simulink library "ESSLibrary"  (R2020a)
settings: Solver=VariableStepAuto  StartTime=0.0  StopTime=10.0  RelTol=1e-3
libraries: $bdroot x82, powerlib_meascontrol x10, simulink x7
(part 6 of 7)

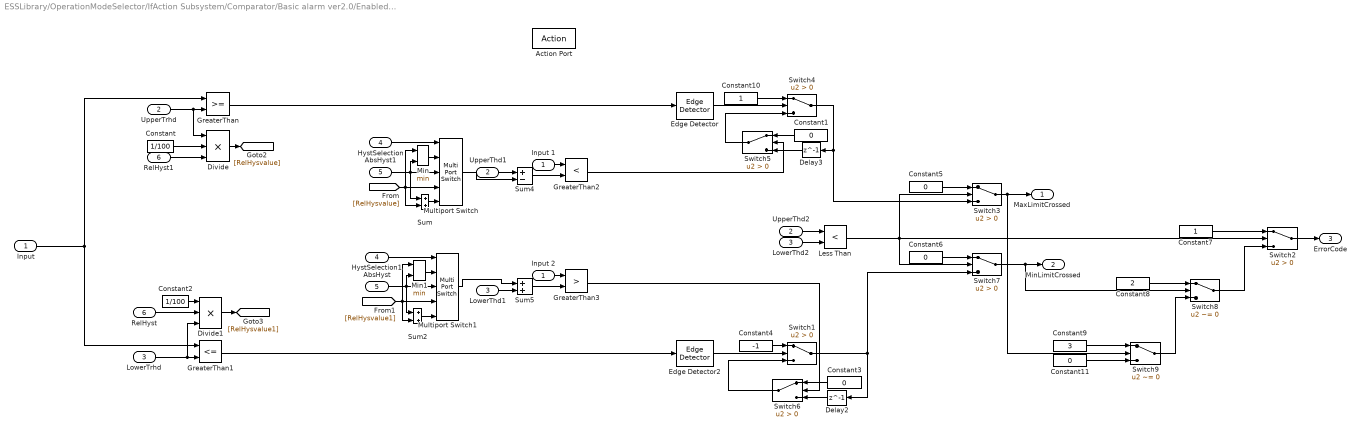
== system ESSLibrary/OperationModeSelector/IfAction Subsystem/Comparator/Basic alarm ver2.0/Enabled Subsystem1 ==
  "Input " : Inport
  UpperTrhd : Inport  Port=2
  LowerTrhd : Inport  Port=3
  HystSelection : Inport  Port=4
  AbsHyst : Inport  Port=5
  RelHyst : Inport  Port=6
  Action Port : ActionPort
  AbsHyst1 : InportShadow  Port=5
  Constant : Constant  Value=1/100  SampleTime=-1
  Constant1 : Constant  Value=0  OutDataTypeStr=int8  SampleTime=-1
  Constant10 : Constant  OutDataTypeStr=int8  SampleTime=-1
  Constant11 : Constant  Value=0  OutDataTypeStr=int64  SampleTime=-1
  Constant2 : Constant  Value=1/100  SampleTime=-1
  Constant3 : Constant  Value=0  OutDataTypeStr=int8  SampleTime=-1
  Constant4 : Constant  Value=-1  OutDataTypeStr=int8  SampleTime=-1
  Constant5 : Constant  Value=0  OutDataTypeStr=boolean  SampleTime=-1
  Constant6 : Constant  Value=0  OutDataTypeStr=boolean  SampleTime=-1
  Constant7 : Constant  OutDataTypeStr=int64  SampleTime=-1
  Constant8 : Constant  Value=2  OutDataTypeStr=int64  SampleTime=-1
  Constant9 : Constant  Value=3  OutDataTypeStr=int64  SampleTime=-1
  Delay2 : Delay  DelayLength=1  InitialCondition=0
  Delay3 : Delay  DelayLength=1  InitialCondition=0
  Divide : Product  Inputs=***
  Divide1 : Product  Inputs=***
  Edge Detector : powerlib_meascontrol/Logic/Edge Detector  model=Rising  ic=0  Ts=-1
      settings: SourceProductBaseCode=PS
  Edge Detector2 : powerlib_meascontrol/Logic/Edge Detector  model=Rising  ic=0  Ts=-1
      settings: SourceProductBaseCode=PS
  GreaterThan : RelationalOperator  OutDataTypeStr=boolean  RndMeth=Simplest
  GreaterThan1 : RelationalOperator  Operator=<=  OutDataTypeStr=boolean  RndMeth=Simplest
  GreaterThan2 : RelationalOperator  Operator=<  OutDataTypeStr=boolean  RndMeth=Simplest
  GreaterThan3 : RelationalOperator  Operator=>  OutDataTypeStr=boolean  RndMeth=Simplest
  HystSelection1 : InportShadow  Port=4
  Input 1 : InportShadow
  Input 2 : InportShadow
  Less Than : RelationalOperator  Operator=<  OutDataTypeStr=boolean  RndMeth=Simplest
  LowerThd1 : InportShadow  Port=3
  LowerThd2 : InportShadow  Port=3
  Min : MinMax  Inputs=2
  Min1 : MinMax  Inputs=2
  Multiport Switch : MultiPortSwitch  Inputs=4
  Multiport Switch1 : MultiPortSwitch  Inputs=4
  RelHyst1 : InportShadow  Port=6
  Sum : Sum
  Sum2 : Sum
  Sum4 : Sum  Inputs=+-
  Sum5 : Sum
  Switch{1..7} (7 alike) : Switch  Criteria=u2 > Threshold
  Switch8 : Switch  Criteria=u2 ~= 0
  Switch9 : Switch  Criteria=u2 ~= 0
  UpperThd1 : InportShadow  Port=2
  UpperThd2 : InportShadow  Port=2
  MaxLimitCrossed : Outport
  MinLimitCrossed : Outport  Port=2
  ErrorCode : Outport  Port=3  OutDataTypeStr=int64
  wires:
  Constant4/1 -> Switch1/1
  GreaterThan/1 -> Edge Detector/1
  "Input "/1 -> GreaterThan/1, GreaterThan1/1
  UpperTrhd/1 -> Divide/1, GreaterThan/2
  LowerTrhd/1 -> Divide1/3, GreaterThan1/2
  HystSelection/1 -> Multiport Switch/1
  AbsHyst1/1 -> Min/2, Sum/1, Multiport Switch/3
  [RelHysvalue] -> Min/1, Sum/2, Multiport Switch/4
  Sum/1 -> Multiport Switch/5
  Divide/1 -> [RelHysvalue]
  Min/1 -> Multiport Switch/2
  Input 1/1 -> GreaterThan2/1
  Constant10/1 -> Switch4/1
  Edge Detector/1 -> Switch4/2
  Switch5/1 -> Switch4/3
  Switch4/1 -> Switch3/3, Delay3/1
  Constant/1 -> Divide/2
  RelHyst1/1 -> Divide/3
  RelHyst/1 -> Divide1/2
  Constant2/1 -> Divide1/1
  Divide1/1 -> [RelHysvalue1]
  HystSelection1/1 -> Multiport Switch1/1
  Min1/1 -> Multiport Switch1/2
  AbsHyst/1 -> Sum2/1, Min1/2, Multiport Switch1/3
  [RelHysvalue1] -> Sum2/2, Multiport Switch1/4, Min1/1
  Sum2/1 -> Multiport Switch1/5
  Input 2/1 -> GreaterThan3/1
  GreaterThan1/1 -> Edge Detector2/1
  Edge Detector2/1 -> Switch1/2
  Switch6/1 -> Switch1/3
  GreaterThan3/1 -> Switch6/2
  Sum4/1 -> GreaterThan2/2
  Multiport Switch/1 -> Sum4/2
  UpperThd1/1 -> Sum4/1
  Sum5/1 -> GreaterThan3/2
  Multiport Switch1/1 -> Sum5/1
  LowerThd1/1 -> Sum5/2
  GreaterThan2/1 -> Switch5/2
  Constant1/1 -> Switch5/1
  Constant3/1 -> Switch6/1
  Delay3/1 -> Switch5/3
  Delay2/1 -> Switch6/3
  Switch3/1 -> Switch9/2, MaxLimitCrossed/1
  Less Than/1 -> Switch2/2, Switch3/2, Switch7/2
  Constant5/1 -> Switch3/1
  Switch1/1 -> Switch7/3, Delay2/1
  Constant6/1 -> Switch7/1
  Switch7/1 -> Switch8/2, MinLimitCrossed/1
  Switch8/1 -> Switch2/3
  Constant7/1 -> Switch2/1
  Switch2/1 -> ErrorCode/1
  LowerThd2/1 -> Less Than/2
  UpperThd2/1 -> Less Than/1
  Constant8/1 -> Switch8/1
  Constant9/1 -> Switch9/1
  Constant11/1 -> Switch9/3
  Switch9/1 -> Switch8/3

== system ESSLibrary/PFReference_P/If Action Subsystem/Safe Divider/Subsystem/Subsystem21 ==
  Denominator : Inport  OutDataTypeStr=double
  Compare To Zero : simulink/Logic and Bit Operations/Compare To Zero  relop===  OutDataTypeStr=boolean
  Constant : Constant  Value=0  SampleTime=-1
  Constant1 : Constant  Value=0  SampleTime=-1
  Constant4 : Constant  Value=1000  SampleTime=-1
  Sum : Sum  Inputs=|++
  Switch1 : Switch  Criteria=u2 > Threshold  Threshold=-0.00001
  Switch2 : Switch  Criteria=u2 > Threshold  Threshold=0.00001
  Switch3 : Switch  Criteria=u2 ~= 0
  Divisor : Outport  OutDataTypeStr=double
  Quality : Outport  Port=2  OutDataTypeStr=boolean
  wires:
  Constant4/1 -> Switch3/3
  Compare To Zero/1 -> Quality/1
  Switch3/1 -> Divisor/1
  Sum/1 -> Compare To Zero/1, Switch3/2, Switch3/1
  Constant/1 -> Switch2/3
  Constant1/1 -> Switch1/1
  Denominator/1 -> Switch2/2, Switch2/1, Switch1/2, Switch1/3
  Switch2/1 -> Sum/1
  Switch1/1 -> Sum/2

== system ESSLibrary/QReference_PF/If Action Subsystem/Subsystem1/Safe Divider/Subsystem ==
  Numerator : Inport  OutDataTypeStr=double
  Denominator : Inport  Port=2  OutDataTypeStr=double
  Action Port : ActionPort
  Constant1 : Constant  OutDataTypeStr=int64  SampleTime=-1
  Constant11 : Constant  SampleTime=-1
  Constant2 : Constant  Value=0  OutDataTypeStr=int64  SampleTime=-1
  Divide8 : Product  Inputs=*/
  NOT : Logic  Operator=NOT  IconShape=distinctive  AllPortsSameDT=off  OutDataTypeStr=boolean
  NOT1 : Logic  Operator=NOT  IconShape=distinctive  AllPortsSameDT=off  OutDataTypeStr=boolean
  Subsystem21 : Subsystem
  Switch1 : Switch  Criteria=u2 ~= 0
  Switch11 : Switch  Criteria=u2 ~= 0
  Quality : Outport  OutDataTypeStr=boolean
  Out : Outport  Port=2  OutDataTypeStr=double
  ErrorCode : Outport  Port=3  OutDataTypeStr=int64
  wires:
  [Quality2] -> Quality/1
  Constant2/1 -> Switch1/1
  Switch11/1 -> Out/1
  Subsystem21/2(Quality) -> [Quality2]
  Constant11/1 -> Switch11/3
  Subsystem21/1(Divisor) -> [Divisor]
  Numerator/1 -> Divide8/1
  Divide8/1 -> Switch11/1
  [Quality2] -> NOT/1
  [Divisor] -> Divide8/2
  Denominator/1 -> Subsystem21/1(Denominator)
  Constant1/1 -> Switch1/3
  Switch1/1 -> ErrorCode/1
  [Quality2] -> NOT1/1
  NOT/1 -> Switch11/2
  NOT1/1 -> Switch1/2

== system ESSLibrary/QReference_PF/If Action Subsystem/Subsystem1/Safe Divider/Subsystem1 ==
  In1 : Inport  OutDataTypeStr=double
  Action Port : ActionPort
  Constant1 : Constant  Value=9  OutDataTypeStr=int64  SampleTime=-1
  Constant11 : Constant  Value=0  OutDataTypeStr=boolean  SampleTime=-1
  Out3 : Outport  OutDataTypeStr=boolean
  Out4 : Outport  Port=2  OutDataTypeStr=double
  Out5 : Outport  Port=3  OutDataTypeStr=int64
  wires:
  Constant1/1 -> Out5/1
  Constant11/1 -> Out3/1
  In1/1 -> Out4/1

== system ESSLibrary/SoCManagement/IfActionSubsystem/Comparator/Basic alarm ver2.0/Enabled Subsystem ==
  Action Port : ActionPort
  Constant3 : Constant  Value=0  OutDataTypeStr=boolean  SampleTime=-1
  "MaxLimitCrossed " : Outport
  ErrorCode : Outport  Port=2
  MinLimitCrossed : Outport  Port=3
  wires:
  Constant3/1 -> "MaxLimitCrossed "/1, MinLimitCrossed/1, ErrorCode/1

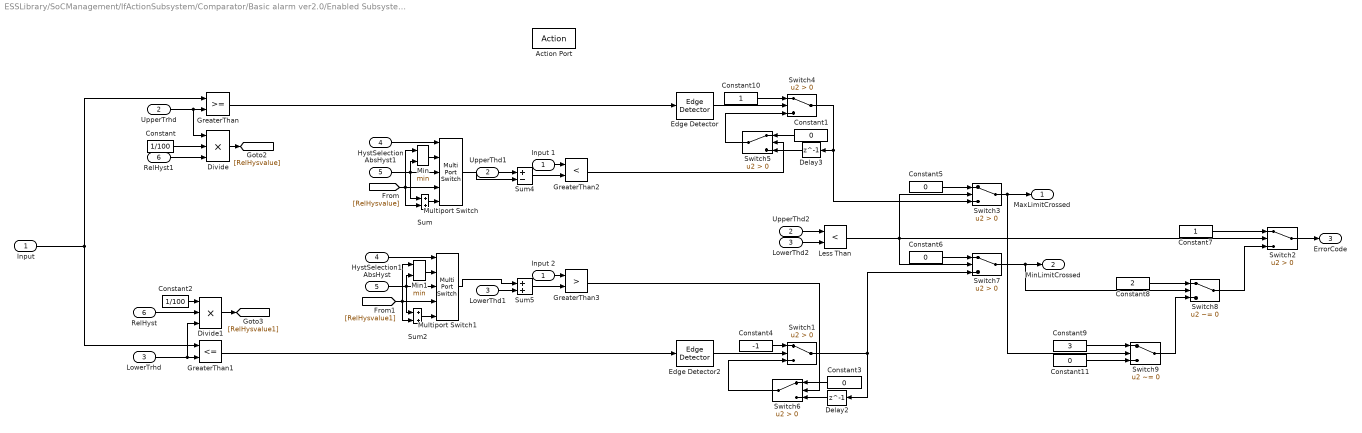
== system ESSLibrary/SoCManagement/IfActionSubsystem/Comparator/Basic alarm ver2.0/Enabled Subsystem1 ==
  "Input " : Inport
  UpperTrhd : Inport  Port=2
  LowerTrhd : Inport  Port=3
  HystSelection : Inport  Port=4
  AbsHyst : Inport  Port=5
  RelHyst : Inport  Port=6
  Action Port : ActionPort
  AbsHyst1 : InportShadow  Port=5
  Constant : Constant  Value=1/100  SampleTime=-1
  Constant1 : Constant  Value=0  OutDataTypeStr=int8  SampleTime=-1
  Constant10 : Constant  OutDataTypeStr=int8  SampleTime=-1
  Constant11 : Constant  Value=0  OutDataTypeStr=int64  SampleTime=-1
  Constant2 : Constant  Value=1/100  SampleTime=-1
  Constant3 : Constant  Value=0  OutDataTypeStr=int8  SampleTime=-1
  Constant4 : Constant  Value=-1  OutDataTypeStr=int8  SampleTime=-1
  Constant5 : Constant  Value=0  OutDataTypeStr=boolean  SampleTime=-1
  Constant6 : Constant  Value=0  OutDataTypeStr=boolean  SampleTime=-1
  Constant7 : Constant  OutDataTypeStr=int64  SampleTime=-1
  Constant8 : Constant  Value=2  OutDataTypeStr=int64  SampleTime=-1
  Constant9 : Constant  Value=3  OutDataTypeStr=int64  SampleTime=-1
  Delay2 : Delay  DelayLength=1  InitialCondition=0
  Delay3 : Delay  DelayLength=1  InitialCondition=0
  Divide : Product  Inputs=***
  Divide1 : Product  Inputs=***
  Edge Detector : powerlib_meascontrol/Logic/Edge Detector  model=Rising  ic=0  Ts=-1
      settings: SourceProductBaseCode=PS
  Edge Detector2 : powerlib_meascontrol/Logic/Edge Detector  model=Rising  ic=0  Ts=-1
      settings: SourceProductBaseCode=PS
  GreaterThan : RelationalOperator  OutDataTypeStr=boolean  RndMeth=Simplest
  GreaterThan1 : RelationalOperator  Operator=<=  OutDataTypeStr=boolean  RndMeth=Simplest
  GreaterThan2 : RelationalOperator  Operator=<  OutDataTypeStr=boolean  RndMeth=Simplest
  GreaterThan3 : RelationalOperator  Operator=>  OutDataTypeStr=boolean  RndMeth=Simplest
  HystSelection1 : InportShadow  Port=4
  Input 1 : InportShadow
  Input 2 : InportShadow
  Less Than : RelationalOperator  Operator=<  OutDataTypeStr=boolean  RndMeth=Simplest
  LowerThd1 : InportShadow  Port=3
  LowerThd2 : InportShadow  Port=3
  Min : MinMax  Inputs=2
  Min1 : MinMax  Inputs=2
  Multiport Switch : MultiPortSwitch  Inputs=4
  Multiport Switch1 : MultiPortSwitch  Inputs=4
  RelHyst1 : InportShadow  Port=6
  Sum : Sum
  Sum2 : Sum
  Sum4 : Sum  Inputs=+-
  Sum5 : Sum
  Switch{1..7} (7 alike) : Switch  Criteria=u2 > Threshold
  Switch8 : Switch  Criteria=u2 ~= 0
  Switch9 : Switch  Criteria=u2 ~= 0
  UpperThd1 : InportShadow  Port=2
  UpperThd2 : InportShadow  Port=2
  MaxLimitCrossed : Outport
  MinLimitCrossed : Outport  Port=2
  ErrorCode : Outport  Port=3  OutDataTypeStr=int64
  wires:
  Switch9/1 -> Switch8/3
  Constant11/1 -> Switch9/3
  Constant9/1 -> Switch9/1
  Constant8/1 -> Switch8/1
  UpperThd2/1 -> Less Than/1
  LowerThd2/1 -> Less Than/2
  Switch2/1 -> ErrorCode/1
  Constant7/1 -> Switch2/1
  Switch8/1 -> Switch2/3
  Switch7/1 -> MinLimitCrossed/1, Switch8/2
  Constant6/1 -> Switch7/1
  Switch1/1 -> Delay2/1, Switch7/3
  Constant5/1 -> Switch3/1
  Less Than/1 -> Switch7/2, Switch3/2, Switch2/2
  Switch3/1 -> MaxLimitCrossed/1, Switch9/2
  Delay2/1 -> Switch6/3
  Delay3/1 -> Switch5/3
  Constant3/1 -> Switch6/1
  Constant1/1 -> Switch5/1
  GreaterThan2/1 -> Switch5/2
  LowerThd1/1 -> Sum5/2
  Multiport Switch1/1 -> Sum5/1
  Sum5/1 -> GreaterThan3/2
  UpperThd1/1 -> Sum4/1
  Multiport Switch/1 -> Sum4/2
  Sum4/1 -> GreaterThan2/2
  GreaterThan3/1 -> Switch6/2
  Switch6/1 -> Switch1/3
  Edge Detector2/1 -> Switch1/2
  GreaterThan1/1 -> Edge Detector2/1
  Input 2/1 -> GreaterThan3/1
  Sum2/1 -> Multiport Switch1/5
  [RelHysvalue1] -> Min1/1, Multiport Switch1/4, Sum2/2
  AbsHyst/1 -> Multiport Switch1/3, Min1/2, Sum2/1
  Min1/1 -> Multiport Switch1/2
  HystSelection1/1 -> Multiport Switch1/1
  Divide1/1 -> [RelHysvalue1]
  Constant2/1 -> Divide1/1
  RelHyst/1 -> Divide1/2
  RelHyst1/1 -> Divide/3
  Constant/1 -> Divide/2
  Switch4/1 -> Delay3/1, Switch3/3
  Switch5/1 -> Switch4/3
  Edge Detector/1 -> Switch4/2
  Constant10/1 -> Switch4/1
  Input 1/1 -> GreaterThan2/1
  Min/1 -> Multiport Switch/2
  Divide/1 -> [RelHysvalue]
  Sum/1 -> Multiport Switch/5
  [RelHysvalue] -> Multiport Switch/4, Sum/2, Min/1
  AbsHyst1/1 -> Multiport Switch/3, Sum/1, Min/2
  HystSelection/1 -> Multiport Switch/1
  LowerTrhd/1 -> GreaterThan1/2, Divide1/3
  UpperTrhd/1 -> GreaterThan/2, Divide/1
  "Input "/1 -> GreaterThan1/1, GreaterThan/1
  GreaterThan/1 -> Edge Detector/1
  Constant4/1 -> Switch1/1

== system ESSLibrary/Dispatch/IfActionSubsystem/PrioritySelector/ActivePowerPriority/ActivePowerPriority_PQCurve/PCapability Calculator ==
  input1 : Inport
  input2 : Inport  Port=2
  input3 : Inport  Port=3
  input4 : Inport  Port=4
  input5 : Inport  Port=5
  input6 : Inport  Port=6
  input7 : Inport  Port=7
  input8 : Inport  Port=8
  Max : MinMax  Function=max  Inputs=8
  Max1 : MinMax  Inputs=8
  Maximum : Outport
  Minimum : Outport  Port=2
  wires:
  Max/1 -> Maximum/1
  input3/1 -> Max1/3, Max/3
  input5/1 -> Max1/5, Max/5
  input8/1 -> Max1/8, Max/8
  input7/1 -> Max1/7, Max/7
  input2/1 -> Max1/2, Max/2
  input6/1 -> Max1/6, Max/6
  input4/1 -> Max1/4, Max/4
  input1/1 -> Max1/1, Max/1
  Max1/1 -> Minimum/1

== system ESSLibrary/Dispatch/IfActionSubsystem/PrioritySelector/ActivePowerPriority/ActivePowerPriority_PQCurve/QCapabilityCalculator ==
  X1 : Inport
  Y1 : Inport  Port=2
  X2 : Inport  Port=3
  Y2 : Inport  Port=4
  X3 : Inport  Port=5
  Y3 : Inport  Port=6
  X4 : Inport  Port=7
  Y4 : Inport  Port=8
  X5 : Inport  Port=9
  Y5 : Inport  Port=10
  X6 : Inport  Port=11
  Y6 : Inport  Port=12
  X7 : Inport  Port=13
  Y7 : Inport  Port=14
  X8 : Inport  Port=15
  Y8 : Inport  Port=16
  input : Inport  Port=17
  QMinCalculator : MATLAB Function  TreatAsAtomicUnit=on
  YMaxCalculator : MATLAB Function  TreatAsAtomicUnit=on
  YMax : Outport
  YMin : Outport  Port=2
  wires:
  QMinCalculator/1(YMin) -> YMin/1
  YMaxCalculator/1(YMax) -> YMax/1
  Y3/1 -> QMinCalculator/6(Y3), YMaxCalculator/6(Y3)
  X3/1 -> QMinCalculator/5(X3), YMaxCalculator/5(X3)
  X4/1 -> QMinCalculator/7(X4), YMaxCalculator/7(X4)
  Y2/1 -> QMinCalculator/4(Y2), YMaxCalculator/4(Y2)
  Y4/1 -> QMinCalculator/8(Y4), YMaxCalculator/8(Y4)
  X2/1 -> QMinCalculator/3(X2), YMaxCalculator/3(X2)
  X5/1 -> QMinCalculator/9(X5), YMaxCalculator/9(X5)
  X1/1 -> QMinCalculator/1(X1), YMaxCalculator/1(X1)
  Y1/1 -> QMinCalculator/2(Y1), YMaxCalculator/2(Y1)
  Y5/1 -> QMinCalculator/10(Y5), YMaxCalculator/10(Y5)
  X6/1 -> QMinCalculator/11(X6), YMaxCalculator/11(X6)
  Y6/1 -> QMinCalculator/12(Y6), YMaxCalculator/12(Y6)
  X7/1 -> QMinCalculator/13(X7), YMaxCalculator/13(X7)
  Y7/1 -> QMinCalculator/14(Y7), YMaxCalculator/14(Y7)
  X8/1 -> QMinCalculator/15(X8), YMaxCalculator/15(X8)
  Y8/1 -> QMinCalculator/16(Y8), YMaxCalculator/16(Y8)
  input/1 -> QMinCalculator/17(input), YMaxCalculator/17(input)

== system ESSLibrary/Dispatch/IfActionSubsystem/PrioritySelector/ReactivePowerPriority/ReactivePowerPriority_PQCurve/QCapability Calculator ==
  input1 : Inport
  input2 : Inport  Port=2
  input3 : Inport  Port=3
  input4 : Inport  Port=4
  input5 : Inport  Port=5
  input6 : Inport  Port=6
  input7 : Inport  Port=7
  input8 : Inport  Port=8
  Max : MinMax  Function=max  Inputs=8
  Max1 : MinMax  Inputs=8
  Maximum : Outport
  Minimum : Outport  Port=2
  wires:
  Max/1 -> Maximum/1
  input3/1 -> Max1/3, Max/3
  input5/1 -> Max1/5, Max/5
  input8/1 -> Max1/8, Max/8
  input7/1 -> Max1/7, Max/7
  input2/1 -> Max1/2, Max/2
  input6/1 -> Max1/6, Max/6
  input4/1 -> Max1/4, Max/4
  input1/1 -> Max1/1, Max/1
  Max1/1 -> Minimum/1

== system ESSLibrary/Dispatch/IfActionSubsystem/PrioritySelector/ReactivePowerPriority/ReactivePowerPriority_PQCurve/QCapabilityCalculator ==
  X1 : Inport
  Y1 : Inport  Port=2
  X2 : Inport  Port=3
  Y2 : Inport  Port=4
  X3 : Inport  Port=5
  Y3 : Inport  Port=6
  X4 : Inport  Port=7
  Y4 : Inport  Port=8
  X5 : Inport  Port=9
  Y5 : Inport  Port=10
  X6 : Inport  Port=11
  Y6 : Inport  Port=12
  X7 : Inport  Port=13
  Y7 : Inport  Port=14
  X8 : Inport  Port=15
  Y8 : Inport  Port=16
  input : Inport  Port=17
  QMinCalculator : MATLAB Function  TreatAsAtomicUnit=on
  YMaxCalculator : MATLAB Function  TreatAsAtomicUnit=on
  YMax : Outport
  YMin : Outport  Port=2
  wires:
  QMinCalculator/1(YMin) -> YMin/1
  YMaxCalculator/1(YMax) -> YMax/1
  Y3/1 -> QMinCalculator/6(Y3), YMaxCalculator/6(Y3)
  X3/1 -> QMinCalculator/5(X3), YMaxCalculator/5(X3)
  X4/1 -> QMinCalculator/7(X4), YMaxCalculator/7(X4)
  Y2/1 -> QMinCalculator/4(Y2), YMaxCalculator/4(Y2)
  Y4/1 -> QMinCalculator/8(Y4), YMaxCalculator/8(Y4)
  X2/1 -> QMinCalculator/3(X2), YMaxCalculator/3(X2)
  X5/1 -> QMinCalculator/9(X5), YMaxCalculator/9(X5)
  X1/1 -> QMinCalculator/1(X1), YMaxCalculator/1(X1)
  Y1/1 -> QMinCalculator/2(Y1), YMaxCalculator/2(Y1)
  Y5/1 -> QMinCalculator/10(Y5), YMaxCalculator/10(Y5)
  X6/1 -> QMinCalculator/11(X6), YMaxCalculator/11(X6)
  Y6/1 -> QMinCalculator/12(Y6), YMaxCalculator/12(Y6)
  X7/1 -> QMinCalculator/13(X7), YMaxCalculator/13(X7)
  Y7/1 -> QMinCalculator/14(Y7), YMaxCalculator/14(Y7)
  X8/1 -> QMinCalculator/15(X8), YMaxCalculator/15(X8)
  Y8/1 -> QMinCalculator/16(Y8), YMaxCalculator/16(Y8)
  input/1 -> QMinCalculator/17(input), YMaxCalculator/17(input)

== system ESSLibrary/QReference_PF/If Action Subsystem/Subsystem1/Safe Divider/Subsystem/Subsystem21 ==
  Denominator : Inport  OutDataTypeStr=double
  Compare To Zero : simulink/Logic and Bit Operations/Compare To Zero  relop===  OutDataTypeStr=boolean
  Constant : Constant  Value=0  SampleTime=-1
  Constant1 : Constant  Value=0  SampleTime=-1
  Constant4 : Constant  Value=1000  SampleTime=-1
  Sum : Sum  Inputs=|++
  Switch1 : Switch  Criteria=u2 > Threshold  Threshold=-0.00001
  Switch2 : Switch  Criteria=u2 > Threshold  Threshold=0.00001
  Switch3 : Switch  Criteria=u2 ~= 0
  Divisor : Outport  OutDataTypeStr=double
  Quality : Outport  Port=2  OutDataTypeStr=boolean
  wires:
  Constant4/1 -> Switch3/3
  Compare To Zero/1 -> Quality/1
  Switch3/1 -> Divisor/1
  Sum/1 -> Compare To Zero/1, Switch3/2, Switch3/1
  Constant/1 -> Switch2/3
  Constant1/1 -> Switch1/1
  Denominator/1 -> Switch2/2, Switch2/1, Switch1/2, Switch1/3
  Switch2/1 -> Sum/1
  Switch1/1 -> Sum/2

== matlab function ESSLibrary/VoltWattMode/MATLAB Function ==
  data: X_In input; Y_Out output; Y_In input; HiStartX input; HiStopX input; HiX_PositiveY_Gradient input; HiX_NegativeY_Gradient input; LoStartX input; LoStopX input; LoX_PositiveY_Gradient input; LoX_NegativeY_Gradient input; StartDelay input; StopDelay input
function Y_Out = FourQuadrantDroop(X_In,Y_In,HiStartX,HiStopX,HiX_PositiveY_Gradient,HiX_NegativeY_Gradient,LoStartX,LoStopX,LoX_PositiveY_Gradient,LoX_NegativeY_Gradient,StartDelay, StopDelay)

persistent  HiXTimeStepStartCounter LoXTimeStepStartCounter TimeStepStopCounter Y_calculated HiXDroopEnable LoXDroopEnable;

if isempty(HiXTimeStepStartCounter)  % Called the first time
    HiXTimeStepStartCounter = 0;      
end
if isempty(HiXTimeStepStartCounter)  % Called the first time
    LoXTimeStepStartCounter = 0;      
end
if isempty(TimeStepStopCounter)  % Called the first time
    TimeStepStopCounter = 0;      
end
if isempty(Y_calculated)  % Called the first time
    Y_calculated = 0.0;      
end
if isempty(HiXDroopEnable)  % Called the first time
    HiXDroopEnable = false;      
end
if isempty(LoXDroopEnable)  % Called the first time
    LoXDroopEnable = false;     
end
if ((X_In > HiStartX) && (X_In < HiStopX) && (HiXDroopEnable == false))
    HiXTimeStepStartCounter = HiXTimeStepStartCounter + 1;
    LoXTimeStepStartCounter = 0;
    TimeStepStopCounter = 0;
end
if ((X_In < LoStartX) && (X_In > LoStopX)&& (LoXDroopEnable == false))
    LoXTimeStepStartCounter = LoXTimeStepStartCounter + 1;
    HiXTimeStepStartCounter = 0;
    TimeStepStopCounter = 0;
end
if ((X_In < HiStartX) && (X_In > LoStartX))
    LoXTimeStepStartCounter = 0;
    HiXTimeStepStartCounter = 0;
    TimeStepStopCounter = TimeStepStopCounter + 1;
end
if (HiXTimeStepStartCounter > StartDelay)
    HiXDroopEnable = true;
    if (Y_In > 0.0)
       Y_calculated = Y_In - ((X_In - HiStartX)*HiX_PositiveY_Gradient);
    elseif (Y_In < 0.0)
       Y_calculated = Y_In - ((X_In - HiStartX)*HiX_NegativeY_Gradient);
    end
elseif (LoXTimeStepStartCounter > StartDelay)
    LoXDroopEnable = true;
    if (Y_In > 0.0)
       Y_calculated = Y_In + ((LoStartX - X_In)*LoX_PositiveY_Gradient);
    elseif (Y_In < 0.0)
       Y_calculated = Y_In + ((LoStartX - X_In)*LoX_NegativeY_Gradient);
    end
else
       Y_calculated = Y_In;
end
if (TimeStepStopCounter > StopDelay)
    HiXDroopEnable = false;
    LoXDroopEnable = false;
    HiXTimeStepStartCounter = 0;
    LoXTimeStepStartCounter = 0;
    TimeStepStopCounter = 0;
end
Y_Out = Y_Calculated;

== matlab function ESSLibrary/FrequencyWattMode/MATLAB Function ==
  data: X_In input; Y_Out output; Y_In input; HiStartX input; HiStopX input; HiX_PositiveY_Gradient input; HiX_NegativeY_Gradient input; LoStartX input; LoStopX input; LoX_PositiveY_Gradient input; LoX_NegativeY_Gradient input; StartDelay input; StopDelay input
function Y_Out = FourQuadrantDroop(X_In,Y_In,HiStartX,HiStopX,HiX_PositiveY_Gradient,HiX_NegativeY_Gradient,LoStartX,LoStopX,LoX_PositiveY_Gradient,LoX_NegativeY_Gradient,StartDelay, StopDelay)

persistent  HiXTimeStepStartCounter LoXTimeStepStartCounter TimeStepStopCounter Y_calculated HiXDroopEnable LoXDroopEnable;

if isempty(HiXTimeStepStartCounter)  % Called the first time
    HiXTimeStepStartCounter = 0;      
end
if isempty(HiXTimeStepStartCounter)  % Called the first time
    LoXTimeStepStartCounter = 0;      
end
if isempty(TimeStepStopCounter)  % Called the first time
    TimeStepStopCounter = 0;      
end
if isempty(Y_calculated)  % Called the first time
    Y_calculated = 0.0;      
end
if isempty(HiXDroopEnable)  % Called the first time
    HiXDroopEnable = false;      
end
if isempty(LoXDroopEnable)  % Called the first time
    LoXDroopEnable = false;     
end
if ((X_In > HiStartX) && (X_In < HiStopX) && (HiXDroopEnable == false))
    HiXTimeStepStartCounter = HiXTimeStepStartCounter + 1;
    LoXTimeStepStartCounter = 0;
    TimeStepStopCounter = 0;
end
if ((X_In < LoStartX) && (X_In > LoStopX)&& (LoXDroopEnable == false))
    LoXTimeStepStartCounter = LoXTimeStepStartCounter + 1;
    HiXTimeStepStartCounter = 0;
    TimeStepStopCounter = 0;
end
if ((X_In < HiStartX) && (X_In > LoStartX))
    LoXTimeStepStartCounter = 0;
    HiXTimeStepStartCounter = 0;
    TimeStepStopCounter = TimeStepStopCounter + 1;
end
if (HiXTimeStepStartCounter > StartDelay)
    HiXDroopEnable = true;
    if (Y_In > 0.0)
       Y_calculated = Y_In - ((X_In - HiStartX)*HiX_PositiveY_Gradient);
    elseif (Y_In < 0.0)
       Y_calculated = Y_In - ((X_In - HiStartX)*HiX_NegativeY_Gradient);
    end
elseif (LoXTimeStepStartCounter > StartDelay)
    LoXDroopEnable = true;
    if (Y_In > 0.0)
       Y_calculated = Y_In + ((LoStartX - X_In)*LoX_PositiveY_Gradient);
    elseif (Y_In < 0.0)
       Y_calculated = Y_In + ((LoStartX - X_In)*LoX_NegativeY_Gradient);
    end
else
       Y_calculated = Y_In;
end
if (TimeStepStopCounter > StopDelay)
    HiXDroopEnable = false;
    LoXDroopEnable = false;
    HiXTimeStepStartCounter = 0;
    LoXTimeStepStartCounter = 0;
    TimeStepStopCounter = 0;
end
Y_Out = Y_Calculated;

== matlab function ESSLibrary/ActivePowerSmoothing/MovAvgDeltaVoltCalc/IfMovAvgFilter/DiscreteMovingAverage ==
  data: NoOfTS input; Out output; Inp input; ErrorCode output
function [Out, ErrorCode] = fcn(NoOfTS,Inp)
% This code generates a moving average filter
NoOfTS = floor(NoOfTS);
ArraySize = 900;
Out = 0;
ErrorCode = 0;
if (NoOfTS > ArraySize)
    ErrorCode = 010102;
    NoOfTS = ArraySize;
end
persistent buffer bufferIndex;
if isempty(buffer)  % Called the first time
    buffer = zeros(NoOfTS,1);
    bufferIndex = 0;  
    for i = 1:1:NoOfTS
    buffer(i)= Inp;
    end
end
bufferIndex         = bufferIndex + 1;
if bufferIndex == (NoOfTS+1)
    bufferIndex         =  1;
end
buffer(bufferIndex) = Inp;
for i = 1:1:NoOfTS
    Out = Out + buffer(i);
end
Out = Out/NoOfTS;

== matlab function ESSLibrary/ActivePowerSmoothing/MATLAB Function ==
  data: X_In input; Y_Out output; X_Ref input; Y_Offset input; X_Hi_Deadband input; X_Lo_Deadband input; X_Hi_Gradient input; X_Lo_Gradient input; StartDelay input; StopDelay input
function Y_Out = TwoQuadrantDroop(X_In,X_Ref,Y_Offset,X_Hi_Deadband,X_Lo_Deadband, X_Hi_Gradient, X_Lo_Gradient,StartDelay, StopDelay)

persistent  HiXTimeStepStartCounter LoXTimeStepStartCounter TimeStepStopCounter Y_calculated HiXDroopEnable LoXDroopEnable;

if isempty(HiXTimeStepStartCounter)  % Called the first time
    HiXTimeStepStartCounter = 0;      
end
if isempty(LoXTimeStepStartCounter)  % Called the first time
    LoXTimeStepStartCounter = 0;      
end
if isempty(TimeStepStopCounter)  % Called the first time
    TimeStepStopCounter = 0;      
end
if isempty(Y_calculated)  % Called the first time
    Y_calculated = 0.0;      
end
if isempty(HiXDroopEnable)  % Called the first time
    HiXDroopEnable = false;      
end
if isempty(LoXDroopEnable)  % Called the first time
    LoXDroopEnable = false;     
end
if ((X_In > (X_Ref + X_Hi_Deadband)) && (HiXDroopEnable == false))
    HiXTimeStepStartCounter = HiXTimeStepStartCounter + 1;
    LoXTimeStepStartCounter = 0;
    TimeStepStopCounter = 0;
end
if ((X_In < (X_Ref - X_Lo_Deadband))&& (LoXDroopEnable == false))
    LoXTimeStepStartCounter = LoXTimeStepStartCounter + 1;
    HiXTimeStepStartCounter = 0;
    TimeStepStopCounter = 0;
end
if ((X_In < (X_Ref + X_Hi_Deadband)) && (X_In > (X_Ref - X_Lo_Deadband)))
    LoXTimeStepStartCounter = 0;
    HiXTimeStepStartCounter = 0;
    TimeStepStopCounter = TimeStepStopCounter + 1;
end
if (HiXTimeStepStartCounter > StartDelay)
    HiXDroopEnable = true;
    
    Y_calculated = Y_Offset - ((X_In - (X_Ref + X_Hi_Deadband)) * X_Hi_Gradient);
    
elseif (LoXTimeStepStartCounter > StartDelay)
    LoXDroopEnable = true;
    
    Y_calculated = Y_Offset + (((X_Ref - X_Lo_Deadband) - X_In) * X_Lo_Gradient);
    
else
    Y_calculated = Y_Offset;
end
if (TimeStepStopCounter > StopDelay)
    HiXDroopEnable = false;
    LoXDroopEnable = false;
    HiXTimeStepStartCounter = 0;
    LoXTimeStepStartCounter = 0;
    TimeStepStopCounter = 0;
end
Y_Out = Y_Calculated;

== matlab function ESSLibrary/DynamicVoltWattMode/MATLAB Function ==
  data: X_In input; Y_Out output; X_Ref input; Y_Offset input; X_Hi_Deadband input; X_Lo_Deadband input; X_Hi_Gradient input; X_Lo_Gradient input; StartDelay input; StopDelay input
function Y_Out = TwoQuadrantDroop(X_In,X_Ref,Y_Offset,X_Hi_Deadband,X_Lo_Deadband, X_Hi_Gradient, X_Lo_Gradient,StartDelay, StopDelay)

persistent  HiXTimeStepStartCounter LoXTimeStepStartCounter TimeStepStopCounter Y_calculated HiXDroopEnable LoXDroopEnable;

if isempty(HiXTimeStepStartCounter)  % Called the first time
    HiXTimeStepStartCounter = 0;      
end
if isempty(LoXTimeStepStartCounter)  % Called the first time
    LoXTimeStepStartCounter = 0;      
end
if isempty(TimeStepStopCounter)  % Called the first time
    TimeStepStopCounter = 0;      
end
if isempty(Y_calculated)  % Called the first time
    Y_calculated = 0.0;      
end
if isempty(HiXDroopEnable)  % Called the first time
    HiXDroopEnable = false;      
end
if isempty(LoXDroopEnable)  % Called the first time
    LoXDroopEnable = false;     
end
if ((X_In > (X_Ref + X_Hi_Deadband)) && (HiXDroopEnable == false))
    HiXTimeStepStartCounter = HiXTimeStepStartCounter + 1;
    LoXTimeStepStartCounter = 0;
    TimeStepStopCounter = 0;
end
if ((X_In < (X_Ref - X_Lo_Deadband))&& (LoXDroopEnable == false))
    LoXTimeStepStartCounter = LoXTimeStepStartCounter + 1;
    HiXTimeStepStartCounter = 0;
    TimeStepStopCounter = 0;
end
if ((X_In < (X_Ref + X_Hi_Deadband)) && (X_In > (X_Ref - X_Lo_Deadband)))
    LoXTimeStepStartCounter = 0;
    HiXTimeStepStartCounter = 0;
    TimeStepStopCounter = TimeStepStopCounter + 1;
end
if (HiXTimeStepStartCounter > StartDelay)
    HiXDroopEnable = true;
    
    Y_calculated = Y_Offset - ((X_In - (X_Ref + X_Hi_Deadband)) * X_Hi_Gradient);
    
elseif (LoXTimeStepStartCounter > StartDelay)
    LoXDroopEnable = true;
    
    Y_calculated = Y_Offset + (((X_Ref - X_Lo_Deadband) - X_In) * X_Lo_Gradient);
    
else
    Y_calculated = Y_Offset;
end
if (TimeStepStopCounter > StopDelay)
    HiXDroopEnable = false;
    LoXDroopEnable = false;
    HiXTimeStepStartCounter = 0;
    LoXTimeStepStartCounter = 0;
    TimeStepStopCounter = 0;
end
Y_Out = Y_Calculated;

== matlab function ESSLibrary/PreProcessing/IfActionSubsystem/3PointAverge ==
  data: Enable input; Out output; Inp1 input; Inp2 input; Inp3 input
function Out = fcn(Enable, Inp1, Inp2, Inp3)
Out = 0.0;
if Enable
    Out = (Inp1+Inp2+Inp3)/3.0;
else
    Out = 0.0;
end

== matlab function ESSLibrary/DynamicVoltWattMode/MovAvgDeltaVoltCalc/IfMovAvgFilter/DiscreteMovingAverage ==
  data: NoOfTS input; Out output; Inp input; ErrorCode output
function [Out, ErrorCode] = fcn(NoOfTS,Inp)
% This code generates a moving average filter
NoOfTS = floor(NoOfTS);
ArraySize = 900;
Out = 0;
ErrorCode = 0;
if (NoOfTS > ArraySize)
    ErrorCode = 010102;
    NoOfTS = ArraySize;
end
persistent buffer bufferIndex;
if isempty(buffer)  % Called the first time
    buffer = zeros(NoOfTS,1);
    bufferIndex = 0;  
    for i = 1:1:NoOfTS
    buffer(i)= Inp;
    end
end
bufferIndex         = bufferIndex + 1;
if bufferIndex == (NoOfTS+1)
    bufferIndex         =  1;
end
buffer(bufferIndex) = Inp;
for i = 1:1:NoOfTS
    Out = Out + buffer(i);
end
Out = Out/NoOfTS;

== matlab function ESSLibrary/WattVarMode/MATLAB Function1 ==
  data: X_In input; X_Hi_Start input; X_Hi_Stop input; X_Lo_Start input; X_Lo_Stop input; X_Hi_Gradient input; X_Lo_Gradient input; Y_Out output; Y_Offset input; StartDelay input; StopDelay input
function Y_Out = TwoQuadrantDroop_PointBased(X_In,X_Hi_Start,X_Hi_Stop, X_Lo_Start, X_Lo_Stop, X_Hi_Gradient, X_Lo_Gradient,Y_Offset,StartDelay, StopDelay)

persistent  HiXTimeStepStartCounter LoXTimeStepStartCounter TimeStepStopCounter Y_calculated HiXDroopEnable LoXDroopEnable;

if isempty(HiXTimeStepStartCounter)  % Called the first time
    HiXTimeStepStartCounter = 0;      
end
if isempty(LoXTimeStepStartCounter)  % Called the first time
    LoXTimeStepStartCounter = 0;      
end
if isempty(TimeStepStopCounter)  % Called the first time
    TimeStepStopCounter = 0;      
end
if isempty(Y_calculated)  % Called the first time
    Y_calculated = 0.0;      
end
if isempty(HiXDroopEnable)  % Called the first time
    HiXDroopEnable = false;      
end
if isempty(LoXDroopEnable)  % Called the first time
    LoXDroopEnable = false;     
end
if ((X_In > X_Hi_Start) && (X_In < X_Hi_Stop) && (HiXDroopEnable == false))
    HiXTimeStepStartCounter = HiXTimeStepStartCounter + 1;
    LoXTimeStepStartCounter = 0;
    TimeStepStopCounter = 0;
end
if ((X_In < X_Lo_Start)&& (X_In > X_Lo_Stop)&& (LoXDroopEnable == false))
    LoXTimeStepStartCounter = LoXTimeStepStartCounter + 1;
    HiXTimeStepStartCounter = 0;
    TimeStepStopCounter = 0;
end
if ((X_In < X_Hi_Start) && (X_In > X_Lo_Start))
    LoXTimeStepStartCounter = 0;
    HiXTimeStepStartCounter = 0;
    TimeStepStopCounter = TimeStepStopCounter + 1;
end
if (HiXTimeStepStartCounter > StartDelay)
    HiXDroopEnable = true;
    
    Y_calculated = Y_Offset - ((X_In - X_Hi_Start) * X_Hi_Gradient);
    
elseif (LoXTimeStepStartCounter > StartDelay)
    LoXDroopEnable = true;
    
    Y_calculated = Y_Offset + ((X_Lo_Start - X_In) * X_Lo_Gradient);
    
else
    Y_calculated = Y_Offset;
end
if (TimeStepStopCounter > StopDelay)
    HiXDroopEnable = false;
    LoXDroopEnable = false;
    HiXTimeStepStartCounter = 0;
    LoXTimeStepStartCounter = 0;
    TimeStepStopCounter = 0;
end
Y_Out = Y_Calculated;

== matlab function ESSLibrary/VoltVarMode/TwoQuadrantDroop_PointBased ==
  data: X_In input; X_Hi_Start input; X_Hi_Stop input; X_Lo_Start input; X_Lo_Stop input; X_Hi_Gradient input; X_Lo_Gradient input; Y_Out output; Y_Offset input; StartDelay input; StopDelay input
function Y_Out = TwoQuadrantDroop_PointBased(X_In,X_Hi_Start,X_Hi_Stop, X_Lo_Start, X_Lo_Stop, X_Hi_Gradient, X_Lo_Gradient,Y_Offset,StartDelay, StopDelay)

persistent  HiXTimeStepStartCounter LoXTimeStepStartCounter TimeStepStopCounter Y_calculated HiXDroopEnable LoXDroopEnable;

if isempty(HiXTimeStepStartCounter)  % Called the first time
    HiXTimeStepStartCounter = 0;      
end
if isempty(LoXTimeStepStartCounter)  % Called the first time
    LoXTimeStepStartCounter = 0;      
end
if isempty(TimeStepStopCounter)  % Called the first time
    TimeStepStopCounter = 0;      
end
if isempty(Y_calculated)  % Called the first time
    Y_calculated = 0.0;      
end
if isempty(HiXDroopEnable)  % Called the first time
    HiXDroopEnable = false;      
end
if isempty(LoXDroopEnable)  % Called the first time
    LoXDroopEnable = false;     
end
if ((X_In > X_Hi_Start) && (X_In < X_Hi_Stop) && (HiXDroopEnable == false))
    HiXTimeStepStartCounter = HiXTimeStepStartCounter + 1;
    LoXTimeStepStartCounter = 0;
    TimeStepStopCounter = 0;
end
if ((X_In < X_Lo_Start)&& (X_In > X_Lo_Stop)&& (LoXDroopEnable == false))
    LoXTimeStepStartCounter = LoXTimeStepStartCounter + 1;
    HiXTimeStepStartCounter = 0;
    TimeStepStopCounter = 0;
end
if ((X_In < X_Hi_Start) && (X_In > X_Lo_Start))
    LoXTimeStepStartCounter = 0;
    HiXTimeStepStartCounter = 0;
    TimeStepStopCounter = TimeStepStopCounter + 1;
end
if (HiXTimeStepStartCounter > StartDelay)
    HiXDroopEnable = true;
    
    Y_calculated = Y_Offset - ((X_In - X_Hi_Start) * X_Hi_Gradient);
    
elseif (LoXTimeStepStartCounter > StartDelay)
    LoXDroopEnable = true;
    
    Y_calculated = Y_Offset + ((X_Lo_Start - X_In) * X_Lo_Gradient);
    
else
    Y_calculated = Y_Offset;
end
if (TimeStepStopCounter > StopDelay)
    HiXDroopEnable = false;
    LoXDroopEnable = false;
    HiXTimeStepStartCounter = 0;
    LoXTimeStepStartCounter = 0;
    TimeStepStopCounter = 0;
end
Y_Out = Y_Calculated;

== matlab function ESSLibrary/Dispatch/IfActionSubsystem/RampLimiter ==
  data: Enable input; RampVal output; RefVal input; ActVal input; RampRateUp input; RampRateDn input; Reset input; RampEnd output; ErrorCode output
function [RampVal,RampEnd, ErrorCode]  = ramplimiter(Enable, RefVal, ActVal, RampRateUp, RampRateDn, Reset)
% ramplimiter is used to rampup or rampdown the actual value to reach the reference value. 
% Enable the function and provide the ramp rates to be applied on actual
% value, the function output the ramp value that gradually reached to the
% reference value.

% The reference value to be achieved by incresing or decreasing the actual
% value using the respective ramp rates, the actual value is basically a
% measurement. One the measured values reached the reference value, the
% funciton rasises an output rampend. If the reset input is raised then the 
% funciton outputs the measured value as it is. Here the reset input can be
% communication quality.

RampVal = 0;
RampEnd = false;
ErrorCode = 0;
if Enable ==1
    if (Reset == 0)
        RefRate = ((RefVal - ActVal));  
        if ((RefRate > 0)&& (RefRate >= RampRateUp))
            RampVal =  ActVal + RampRateUp;
            ErrorCode = 0;
       
        elseif ((RefRate < 0)&& (RefRate <= -RampRateDn))
            RampVal =   ActVal - RampRateDn;
            ErrorCode = 0;
            
        else
            RampEnd = true;
            RampVal = RefVal;
            ErrorCode = 0;
        end
    end
    if (Reset == 1)
        RampVal = ActVal; 
        ErrorCode = 0;
    end
end

if Enable == 0
    RampVal = ActVal; 
    RampEnd = true; 
    ErrorCode = 0;
end
end

== matlab function ESSLibrary/RampLimiter ==
  data: Enable input; RampVal output; RefVal input; ActVal input; RampRateUp input; RampRateDn input; Reset input; RampEnd output; ErrorCode output
function [RampVal,RampEnd, ErrorCode]  = ramplimiter(Enable, RefVal, ActVal, RampRateUp, RampRateDn, Reset)
% ramplimiter is used to rampup or rampdown the actual value to reach the reference value. 
% Enable the function and provide the ramp rates to be applied on actual
% value, the function output the ramp value that gradually reached to the
% reference value.

% The reference value to be achieved by incresing or decreasing the actual
% value using the respective ramp rates, the actual value is basically a
% measurement. One the measured values reached the reference value, the
% funciton rasises an output rampend. If the reset input is raised then the 
% funciton outputs the measured value as it is. Here the reset input can be
% communication quality.

RampVal = 0;
RampEnd = false;
ErrorCode = 0;
if Enable ==1
    if (Reset == 0)
        RefRate = ((RefVal - ActVal));  
        if ((RefRate > 0)&& (RefRate >= RampRateUp))
            RampVal =  ActVal + RampRateUp;
            ErrorCode = 0;
       
        elseif ((RefRate < 0)&& (RefRate <= -RampRateDn))
            RampVal =   ActVal - RampRateDn;
            ErrorCode = 0;
            
        else
            RampEnd = true;
            RampVal = RefVal;
            ErrorCode = 0;
        end
    end
    if (Reset == 1)
        RampVal = ActVal; 
        ErrorCode = 0;
    end
end

if Enable == 0
    RampVal = ActVal; 
    RampEnd = true; 
    ErrorCode = 0;
end
end

== matlab function ESSLibrary/Dispatch/IfActionSubsystem/PrioritySelector/ActivePowerPriority/ActivePowerPriority_NoPQCurve/ActivePowerPriority_NoPQCurve ==
  data: ActivePowerCalc input; ReactivePowerCalc input; ActivePowerOut output; ECPAppPow input; EnablePFLimit input; PFOperMax input; PFOperMin input; ReactivePowerOut output
function [ActivePowerOut, ReactivePowerOut] = ActivePowerPriority_NoPQCurve(ActivePowerCalc,ReactivePowerCalc,ECPAppPow, EnablePFLimit,PFOperMax,PFOperMin)

if (ActivePowerCalc >= 0.0)
    if(ActivePowerCalc >= ECPAppPow)
        ActivePowerOut = ECPAppPow;
        ReactivePowerOut = 0.0;
    else
        ActivePowerOut = ActivePowerCalc;
        if (EnablePFLimit)
            if (ReactivePowerCalc > 0.0)
                ReactivePowerOut = min(ReactivePowerCalc, (ActivePowerOut/PFOperMax)*sqrt(1 - power(PFOperMax,2)));
            elseif (ReactivePowerCalc < 0.0)
                ReactivePowerOut = max( ReactivePowerCalc, (ActivePowerOut/PFOperMin)*sqrt(1 - power(PFOperMin,2)));
            else
                ReactivePowerOut =0.0;
            end
        else
            if (ReactivePowerCalc > 0.0)
                ReactivePowerOut = min(ReactivePowerCalc, sqrt(power(ECPAppPow,2)-power(ActivePowerOut,2)));
            elseif (ReactivePowerCalc < 0.0)
                ReactivePowerOut = max(ReactivePowerCalc, -1*sqrt(power(ECPAppPow,2)-power(ActivePowerOut,2)));
            else
                ReactivePowerOut =0.0;
            end
        end
    end
elseif (ActivePowerCalc < 0.0)
    ActivePowerCalc = abs(ActivePowerCalc);
    if(ActivePowerCalc >= ECPAppPow)
        ActivePowerOut = -1*ECPAppPow;
        ReactivePowerOut = 0.0;
    else
        ActivePowerOut = -1 * ActivePowerCalc;
        if (EnablePFLimit)
            if (ReactivePowerCalc > 0.0)
                ReactivePowerOut = min(ReactivePowerCalc, (ActivePowerOut/PFOperMin)*sqrt(1 - power(PFOperMin,2)));
            elseif (ReactivePowerCalc < 0.0)
                ReactivePowerOut = max( ReactivePowerCalc, (ActivePowerCalc/PFOperMax)*sqrt(1 - power(PFOperMax,2)));
            else
                ReactivePowerOut =0.0;
            end
        else
            if (ReactivePowerCalc > 0.0)
                ReactivePowerOut = min(ReactivePowerCalc, sqrt(power(ECPAppPow,2)-power(ActivePowerOut,2)));
            elseif (ReactivePowerCalc < 0.0)
                ReactivePowerOut = max(ReactivePowerCalc, -1*sqrt(power(ECPAppPow,2)-power(ActivePowerOut,2)));
            else
                ReactivePowerOut =0.0;
            end
        end
    end    
end

== matlab function ESSLibrary/Dispatch/IfActionSubsystem/PrioritySelector/ActivePowerPriority/ActivePowerPriority_PQCurve/QCapabilityCalculator/YMaxCalculator ==
  data: X1 input; YMax output; Y1 input; X2 input; Y2 input; X3 input; Y3 input; X4 input; Y4 input; X5 input; Y5 input; X6 input; Y6 input; X7 input; Y7 input; X8 input; Y8 input; input input
function YMax      = fcn(X1,Y1,X2,Y2,X3,Y3,X4,Y4,X5,Y5,X6,Y6,X7,Y7,X8,Y8,input)

    XY = [X1 Y1 X2 Y2 X3 Y3 X4 Y4 X5 Y5 X6 Y6 X7 Y7 X8 Y8];

    [~,c] = size(PQ);

    YMax = 0;
    Y_positive = zeros(8,1);
    X_Ypositive= zeros(8,1);
    count = 1;

    for j = 2:2:c
        if XY(1,j) >=0
        Y_positive(count,1)= XY(1,j);
        X_Ypositive(count,1)= XY(1,j-1);
        count =count+1;
        end
    end

    if (count > 2)
        for i = 1:1:(count - 2)
            for j = i+1:1:(count-1)
                if(X_Ypositive(j,1) < X_Ypositive(i,1))
                    a=X_Ypositive(j,1);
                    X_Ypositive(j,1) = X_Ypositive(i,1);
                    X_Ypositive(i,1) = a;
                    a=Y_positive(j,1);
                    Y_positive(j,1) = Y_positive(i,1);
                    Y_positive(i,1) = a;
                end
            end
        end

        for i = 1 :1 : (count - 2)
           if ((input >= X_Ypositive(i,1)) && (input < X_Ypositive(i+1,1)))
               YMax = (((Y_positive(i+1,1)- Y_positive(i,1))/(X_Ypositive(i+1,1)- X_Ypositive(i,1)))* (input - X_Ypositive(i,1)))+ Y_positive(i,1);
               break;
           end
        end
    end
    if (input < X_Ypositive(1,1))
        YMax = Y_positive(1,1);
    end
    if (count > 1) 
        if (input >= X_Ypositive(count-1,1))
            YMax = Y_positive(count-1,1);
        end
    end

end

== matlab function ESSLibrary/Dispatch/IfActionSubsystem/PrioritySelector/ActivePowerPriority/ActivePowerPriority_PQCurve/QCapabilityCalculator/QMinCalculator ==
  data: X1 input; YMin output; Y1 input; X2 input; Y2 input; X3 input; Y3 input; X4 input; Y4 input; X5 input; Y5 input; X6 input; Y6 input; X7 input; Y7 input; X8 input; Y8 input; input input
function YMin     = fcn(X1,Y1,X2,Y2,X3,Y3,X4,Y4,X5,Y5,X6,Y6,X7,Y7,X8,Y8,input)

    XY = [X1 Y1 X2 Y2 X3 Y3 X4 Y4 X5 Y5 X6 Y6 X7 Y7 X8 Y8];

    [~,c] = size(PQ);

    YMin = 0;
    Y_negative = zeros(8,1);
    X_Ynegative = zeros(8,1);
    count = 1;
    for j = 2:2:c
        if XY(1,j) <=0
        Y_negative(count,1)= XY(1,j);
        X_Ynegative(count,1)= XY(1,j-1);
        count =count+1;
        end
    end

    if (count > 2)
        for i = 1:1:(count - 2)
            for j = i+1:1:(count-1)
                if(X_Ynegative(j,1) < X_Ynegative(i,1))
                    a=X_Ynegative(j,1);
                    X_Ynegative(j,1) = X_Ynegative(i,1);
                    X_Ynegative(i,1) = a;
                    a=Y_negative(j,1);
                    Y_negative(j,1) = Y_negative(i,1);
                    Y_negative(i,1) = a;
                end
            end
        end
        for i = 1 :1 : (count - 2)
           if ((input >= X_Ynegative(i,1)) && (input < X_Ynegative(i+1,1)))
               YMin = (((Y_negative(i+1,1)- Y_negative(i,1))/(X_Ynegative(i+1,1)- X_Ynegative(i,1)))* (input - X_Ynegative(i,1)))+ Y_negative(i,1);
           end
        end
    end
    if (input < X_Ynegative(1,1))
        YMin = Y_negative(1,1);
    end
    if (count > 1)
        if (input >= X_Ynegative(count-1,1))
            YMin = Y_negative(count-1);
        end
    end

end

== matlab function ESSLibrary/Dispatch/IfActionSubsystem/PrioritySelector/ActivePowerPriority/ActivePowerPriority_PQCurve/ActivePowerEvaluator ==
  data: ActivePowerCalc input; MaxP_PQCurve input; ActivePowerOut output; MinP_PQCurve input; ECPAppPow input
function ActivePowerOut = ActivePowerEvaluator(ActivePowerCalc, MaxP_PQCurve, MinP_PQCurve, ECPAppPow)
PPositiveLimit =0.0;
PNegativeLimit = 0.0;
if (ActivePowerCalc >= 0.0)
    if (MaxP_PQCurve >= ECPAppPow)
        PPositiveLimit = ECPAppPow;
    else
        PPositiveLimit = MaxP_PQCurve;
    end
    if (ActivePowerCalc >= PPositiveLimit)
        ActivePowerOut = PPositiveLimit;
    else
        ActivePowerOut = ActivePowerCalc;
    end
else
    if (MinP_PQCurve <=  (-1 *ECPAppPow))
        PNegativeLimit = (-1 *ECPAppPow);
    else
        PNegativeLimit = MinP_PQCurve;
    end
    if (ActivePowerCalc <= PNegativeLimit)
        ActivePowerOut = PNegativeLimit;
    else
        ActivePowerOut = ActivePowerCalc;
    end
    
end

== matlab function ESSLibrary/Dispatch/IfActionSubsystem/PrioritySelector/ActivePowerPriority/ActivePowerPriority_PQCurve/ReactivePowerEvaluator ==
  data: ReactivePowerCalc input; ReactivePowerOut output; ActivePowerCalc input; MaxQ_PQCurve input; MinQ_PQCurve input; ECPAppPow input; EnablePFLimit input; PFOperMax input; PFOperMin input
function ReactivePowerOut = ReactivePowerEvaluator(ReactivePowerCalc, ActivePowerCalc, MaxQ_PQCurve, MinQ_PQCurve, ECPAppPow, EnablePFLimit, PFOperMax, PFOperMin)
QPositiveLimit = 0.0;
QPositivePFLimit = 0.0;
QNegativeLimit = 0.0;
QNegativePFLimit = 0.0;
if (ReactivePowerCalc >= 0.0)
    if (MaxQ_PQCurve >= sqrt(power(ECPAppPow,2)- power(ActivePowerCalc,2)))
        QPositiveLimit = sqrt(power(ECPAppPow,2)- power(ActivePowerCalc,2));
    else
        QPositiveLimit = MaxQ_PQCurve;
    end
    if (EnablePFLimit)
        if (ActivePowerCalc >= 0.0)
            QPositivePFLimit = (ActivePowerOut/PFOperMax)*sqrt(1 - power(PFOperMax,2));
        else
            QPositivePFLimit = (ActivePowerOut/PFOperMin)*sqrt(1 - power(PFOperMin,2));
        end
    
        if (ReactivePowerCalc >= min(QPositiveLimit, QPositivePFLimit))
            ReactivePowerOut = min(QPositiveLimit, QPositivePFLimit);
        else
            ReactivePowerOut = ReactivePowerCalc;
        end
    else
        if (ReactivePowerCalc >= QPositiveLimit)
            ReactivePowerOut = QPositiveLimit;
        else
            ReactivePowerOut = ReactivePowerCalc;
        end
    end
    
else
    if (MinQ_PQCurve <= (-1*sqrt(power(ECPAppPow,2)- power(ActivePowerCalc,2))))
        QNegativeLimit = (-1*sqrt(power(ECPAppPow,2)- power(ActivePowerCalc,2)));
    else
        QNegativeLimit = MaxQ_PQCurve;
    end
    if (EnablePFLimit)
        if (ActivePowerCalc >= 0.0)
            QNegativePFLimit = (ActivePowerOut/PFOperMin)*sqrt(1 - power(PFOperMin,2));
        else
            QNegativePFLimit = (ActivePowerOut/PFOperMax)*sqrt(1 - power(PFOperMax,2));
        end
    
        if (ReactivePowerCalc <= min(QNegativeLimit, QNegativePFLimit))
            ReactivePowerOut = min(QNegativeLimit, QNegativePFLimit);
        else
            ReactivePowerOut = ReactivePowerCalc;
        end
    else
        if (ReactivePowerCalc <= QNegativeLimit)
            ReactivePowerOut = QNegativeLimit;
        else
            ReactivePowerOut = ReactivePowerCalc;
        end
    end
    
end

== matlab function ESSLibrary/Dispatch/IfActionSubsystem/PrioritySelector/ReactivePowerPriority/ReactivePowerPriority_NoPQCurve/ReactivePowerPriority_NoPQCurve ==
  data: ActivePowerCalc input; ReactivePowerCalc input; ActivePowerOut output; ECPAppPow input; EnablePFLimit input; PFOperMax input; PFOperMin input; ReactivePowerOut output
function [ActivePowerOut, ReactivePowerOut] = ReactivePowerPriority_NoPQCurve(ActivePowerCalc,ReactivePowerCalc,ECPAppPow, EnablePFLimit,PFOperMax,PFOperMin)

if (ReactivePowerCalc >= 0.0)
    if(ReactivePowerCalc >= ECPAppPow)
        ActivePowerOut = 0.0;
        ReactivePowerOut = ECPAppPow;
    else
        ReactivePowerOut = ReactivePowerCalc;
        if (EnablePFLimit)
            if (ActivePowerCalc > 0.0)
                ActivePowerOut = min(ActivePowerCalc, (ReactivePowerOut*PFOperMax)/sqrt(1 - power(PFOperMax,2)));
            elseif (ActivePowerCalc < 0.0)
                ActivePowerOut = max(ActivePowerCalc, (ReactivePowerOut*PFOperMin)/sqrt(1 - power(PFOperMin,2)));
            else
                ActivePowerOut =0.0;
            end
        else
            if (ActivePowerCalc > 0.0)
                ActivePowerOut = min(ActivePowerCalc, sqrt(power(ECPAppPow,2)-power(ReactivePowerOut,2)));
            elseif (ReactivePowerCalc < 0.0)
                ActivePowerOut = max(ActivePowerCalc, -1*sqrt(power(ECPAppPow,2)-power(ReactivePowerOut,2)));
            else
                ActivePowerOut =0.0;
            end
        end
    end
elseif (ReactivePowerCalc < 0.0)
    ReactivePowerCalc = abs(ReactivePowerCalc);
    if(ReactivePowerCalc >= ECPAppPow)
        ReactivePowerOut = -1*ECPAppPow;
        ActivePowerOut = 0.0;
    else
        ReactivePowerOut = -1 * ActivePowerCalc;
        if (EnablePFLimit)
            if (ActivePowerCalc > 0.0)
                ActivePowerOut = min(ActivePowerCalc, (ReactivePowerOut*PFOperMin)/sqrt(1 - power(PFOperMin,2)));
            elseif (ActivePowerCalc < 0.0)
                ActivePowerOut = max(ActivePowerCalc, (ReactivePowerCalc*PFOperMax)/sqrt(1 - power(PFOperMax,2)));
            else
                ActivePowerOut =0.0;
            end
        else
            if (ActivePowerCalc > 0.0)
                ActivePowerOut = min(ActivePowerCalc, sqrt(power(ECPAppPow,2)-power(ReactivePowerOut,2)));
            elseif (ActivePowerCalc < 0.0)
                ActivePowerOut = max(ActivePowerCalc, -1*sqrt(power(ECPAppPow,2)-power(ReactivePowerOut,2)));
            else
                ActivePowerOut =0.0;
            end
        end
    end    
end
